simulink model "LR5_graph_2"  (R2018a)
settings: Solver=ode45  StartTime=0.0  StopTime=20  RelTol=1e-3  EnableMultiTasking=on
settings Model: Creator=stud507ikt  LastModifiedBy=Asus
settings DataIOCC: LimitDataPoints=on  SaveFormat=Array
settings OptimizationCC: LifeSpan=inf
settings DebuggingCC: SolverPrmCheckMsg=warning  SFUnexpectedBacktrackingDiag=warning  SFNoUnconditionalDefaultTransitionDiag=warning  SFExecutionAtInitializationDiag=none
settings HardwareCC: ProdBitPerPointer=32  ProdBitPerSizeT=32  ProdBitPerPtrDiffT=32  ProdLargestAtomicFloat=None  ProdIntDivRoundTo=Undefined  ProdEndianess=Unspecified  ProdWordSize=32  ProdHWDeviceType=32-bit Generic
settings ModelReferenceCC: PropagateSignalLabelsOutOfModel=off
settings CodeAppCC: StateflowObjectComments=on
settings GRTTargetCC: TargetLangStandard=C89/C90 (ANSI)  GeneratePreprocessorConditionals=Disable all
settings ConfigComp: CovMetricSettings=dw  CovHtmlReporting=on  CovSaveCumulativeToWorkspaceVar=on  CovSaveSingleToWorkspaceVar=on  CovExternalEMLEnable=off  CovSFcnEnable=off

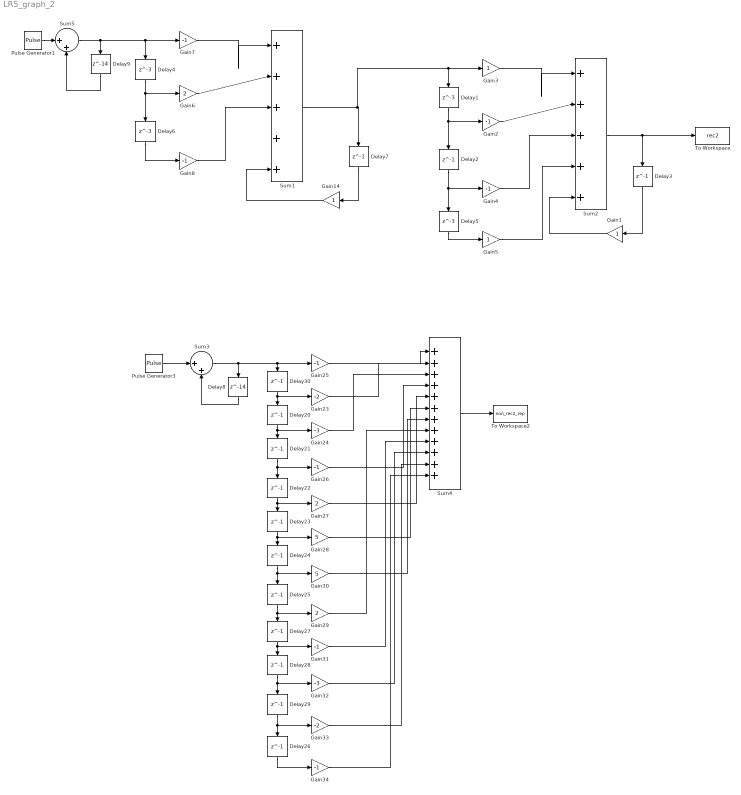
== system LR5_graph_2 ==
  Delay{1,4..6} (4 alike) : Delay  DelayLength=3  InitialCondition=0  InputProcessing=Inherited
  Delay{2..3,7,20..30} (14 alike) : Delay  DelayLength=1  InitialCondition=0  InputProcessing=Inherited
  Delay8 : Delay  DelayLength=14  InitialCondition=0  InputProcessing=Inherited
  Delay9 : Delay  DelayLength=14  InitialCondition=0  InputProcessing=Inherited
  Gain{1,3,5,14} (4 alike) : Gain
  Gain{2,4,7..8,25..26,31,34} (8 alike) : Gain  Gain=-1
  Gain23 : Gain  Gain=-2
  Gain24 : Gain  Gain=-3
  Gain27 : Gain  Gain=2
  Gain28 : Gain  Gain=5
  Gain29 : Gain  Gain=2
  Gain30 : Gain  Gain=5
  Gain32 : Gain  Gain=-3
  Gain33 : Gain  Gain=-2
  Gain6 : Gain  Gain=2
  Pulse Generator1 : DiscretePulseGenerator  Period=10000
  Pulse Generator3 : DiscretePulseGenerator  Period=10000
  Sum1 : Sum  Inputs=|+++++
  Sum2 : Sum  Inputs=|+++++
  Sum3 : Sum  Inputs=|++
  Sum4 : Sum  Inputs=|++++++++++++
  Sum5 : Sum  Inputs=|++
  To Workspace : ToWorkspace  VariableName=rec2  SampleTime=-1
  To Workspace2 : ToWorkspace  VariableName=non_rec2_rep  SampleTime=-1
  wires:
  Gain6/1 -> Sum1/2
  Gain7/1 -> Sum1/1
  Gain8/1 -> Sum1/3
  Delay6/1 -> Gain8/1
  Delay7/1 -> Gain14/1
  Delay4/1 -> Delay6/1, Gain6/1
  Gain14/1 -> Sum1/5
  Gain2/1 -> Sum2/2
  Gain3/1 -> Sum2/1
  Gain4/1 -> Sum2/3
  Delay2/1 -> Delay5/1, Gain4/1
  Delay5/1 -> Gain5/1
  Gain5/1 -> Sum2/4
  Sum1/1 -> Gain3/1, Delay1/1, Delay7/1
  Delay3/1 -> Gain1/1
  Delay1/1 -> Delay2/1, Gain2/1
  Sum2/1 -> To Workspace/1, Delay3/1
  Gain1/1 -> Sum2/5
  Gain28/1 -> Sum4/6
  Gain34/1 -> Sum4/12
  Gain29/1 -> Sum4/8
  Gain30/1 -> Sum4/7
  Gain23/1 -> Sum4/2
  Delay23/1 -> Gain28/1, Delay24/1
  Delay22/1 -> Gain27/1, Delay23/1
  Gain33/1 -> Sum4/11
  Delay25/1 -> Gain29/1, Delay27/1
  Gain27/1 -> Sum4/5
  Delay24/1 -> Gain30/1, Delay25/1
  Gain32/1 -> Sum4/10
  Sum4/1 -> To Workspace2/1
  Delay21/1 -> Gain26/1, Delay22/1
  Delay26/1 -> Gain34/1
  Gain26/1 -> Sum4/4
  Delay29/1 -> Delay26/1, Gain33/1
  Gain25/1 -> Sum4/1
  Delay28/1 -> Gain32/1, Delay29/1
  Gain31/1 -> Sum4/9
  Delay20/1 -> Gain24/1, Delay21/1
  Delay27/1 -> Gain31/1, Delay28/1
  Gain24/1 -> Sum4/3
  Delay30/1 -> Gain23/1, Delay20/1
  Pulse Generator3/1 -> Sum3/1
  Sum3/1 -> Delay8/1, Delay30/1, Gain25/1
  Delay8/1 -> Sum3/2
  Delay9/1 -> Sum5/2
  Sum5/1 -> Delay4/1, Gain7/1, Delay9/1
  Pulse Generator1/1 -> Sum5/1
